simulink model "ControleSimplificado"  (R2018b)
settings: Solver=VariableStepAuto  StartTime=0.0  StopTime=30  RelTol=1e-3
values from neighbouring files (symbols this model uses):
  C = [0 0 0 0 1 0 0 0 0 0 0 0 ... (first row only)    [ControleSimplificado.m]    (also in Plano_Piloto_trabalho.m = [1 0 0 0 0 0 0 0 0 0 0 0)
  Dk = D    [ControleSimplificado.m]    (also in Plano_Piloto_trabalho.m)
  G = expm(A*T)    [ControleSimplificado.m]    (also in Plano_Piloto_trabalho.m = eye(12) + A*T)
  Gravidade = [0 ... (first row only)    [ControleSimplificado.m]
  H = double(H)    [ControleSimplificado.m]    (also in Plano_Piloto_trabalho.m = T*B)
  Rv = 1e-9*diag([1 1 1 1])    [ControleSimplificado.m]
  T = 0.01    [ControleSimplificado.m]    (also in Plano_Piloto_trabalho.m)
undefined symbols (not defined in the file or in its folder): Discrete, K, Time
libraries: ctrlSharedLib x1
settings Model: Creator=Adm  LastModifiedBy=Adm

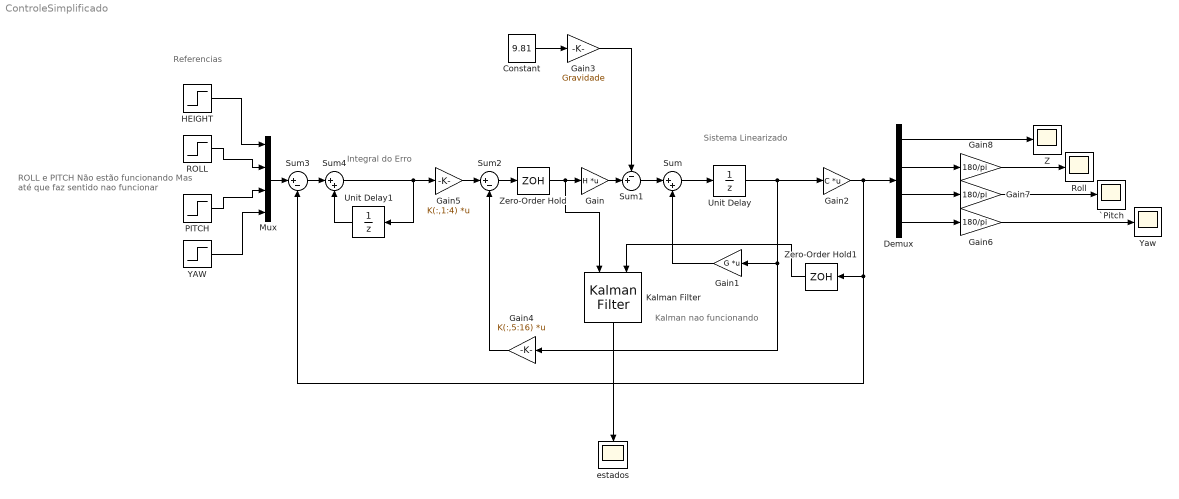
== system ControleSimplificado ==
  note: Kalman nao funcionando
  note: ROLL e PITCH
      | Não estão funcionando
      | Mas até que faz sentido nao funcionar
  note: Referencias
  note: Integral do Erro
  note: Sistema Linearizado
  Constant : Constant  Value=9.81
  Demux : Demux
  Gain : Gain  Gain=H  Multiplication=Matrix(K*u)
  Gain1 : Gain  Gain=G  Multiplication=Matrix(K*u)
  Gain2 : Gain  Gain=C  Multiplication=Matrix(K*u)
  Gain3 : Gain  Gain=Gravidade
  Gain4 : Gain  Gain=K(:,5:16)  Multiplication=Matrix(K*u)
  Gain5 : Gain  Gain=K(:,1:4)  Multiplication=Matrix(K*u)
  Gain6 : Gain  Gain=180/pi
  Gain7 : Gain  Gain=180/pi
  Gain8 : Gain  Gain=180/pi
  HEIGHT : Step  After=-5  SampleTime=0
  Kalman Filter : ctrlSharedLib/Kalman Filter  TimeDomain=Discrete-Time  UseCurrentEstimator=on  ModelSource=LTI State-Space Variable  ModelSourceVariable=sysD  A=G  B=H  C=C  D=Dk  NumberOfStates=1  NumberOfInputs=1  NumberOfOutputs=1  InitialEstimateSource=Dialog  X0=0  P0=10  UseK=off  UseGH=off  NumberOfProcessNoiseInputs=1  G=1  TimeInvariantG=on  H=0  TimeInvariantH=on  Q=Qw  TimeInvariantQ=on  R=Rv  TimeInvariantR=on  N=0  TimeInvariantN=on  AddInputPort=on  AddEnablePort=off  OutputEstimatedY=off  OutputP=off  Ts=T
      settings: SourceProductBaseCode=CT
  Mux : Mux
  PITCH : Step  After=0  SampleTime=0
  ROLL : Step  After=25*pi/180  SampleTime=0
  Roll : Scope
  Sum : Sum  Inputs=|++
  Sum1 : Sum  Inputs=-+|
  Sum2 : Sum  Inputs=|+-
  Sum3 : Sum  Inputs=|+-
  Sum4 : Sum  Inputs=|++
  Unit Delay : UnitDelay  SampleTime=T
  Unit Delay1 : UnitDelay  SampleTime=T
  YAW : Step  After=25*pi/180  SampleTime=0
  Yaw : Scope
  Z : Scope
  Zero-Order Hold : ZeroOrderHold  SampleTime=T
  Zero-Order Hold1 : ZeroOrderHold  SampleTime=T
  `Pitch : Scope
  estados : Scope
  wires:
  Gain3/1 -> Sum1/1
  PITCH/1 -> Mux/3
  Sum1/1 -> Sum/1
  Gain/1 -> Sum1/2
  YAW/1 -> Mux/4
  Constant/1 -> Gain3/1
  Unit Delay/1 -> Gain2/1, Gain4/1, Gain1/1
  Sum/1 -> Unit Delay/1
  Gain1/1 -> Sum/2
  Zero-Order Hold/1 -> Kalman Filter/1, Gain/1
  ROLL/1 -> Mux/2
  HEIGHT/1 -> Mux/1
  Sum2/1 -> Zero-Order Hold/1
  Gain4/1 -> Sum2/2
  Mux/1 -> Sum3/1
  Gain5/1 -> Sum2/1
  Sum3/1 -> Sum4/1
  Sum4/1 -> Unit Delay1/1, Gain5/1
  Unit Delay1/1 -> Sum4/2
  Demux/1 -> Z/1
  Kalman Filter/1 -> estados/1
  Gain2/1 -> Demux/1, Zero-Order Hold1/1, Sum3/2
  Zero-Order Hold1/1 -> Kalman Filter/2
  Demux/4 -> Gain6/1
  Gain6/1 -> Yaw/1
  Gain7/1 -> `Pitch/1
  Demux/3 -> Gain7/1
  Demux/2 -> Gain8/1
  Gain8/1 -> Roll/1
